simulink library "Ventilation_AIV"  (Simulink 8.2)
settings: Solver=ode45  StartTime=0.0  StopTime=10.0  RelTol=1e-3
libraries: carnot x3
settings Model: Creator=lena.frank  LastModifiedBy=drhf

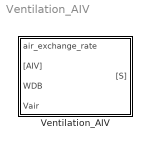
== system Ventilation_AIV ==
  Ventilation_AIV : Subsystem  mask(ACTIVE COMPONENT){co2=400}
      mask prompts: co2 "CO2 content of air in ppm"
      mask help:
      | This block represents the AIR VENTILATION from outdoors into a zone.
      |
      | r : rate of nominal air flow between outdoors and indoor, [0,1]
      | [S] : vector for sinks and sources.
      |
      | NOTE: Mass flows of water and CO2 are taken into consideration.
      |
      | ASSUMPTION:
      | Incoming air volume flow is identical to outgoing air volume flow.
      mask init:
      | CO2norm = co2*1e-6;
      mask Help: web(fullfile(path_carnot('help'),'Ventilation_AIV.html'),'-helpbrowser')
      mask Display:
      | plot([0.2 0.35], [0.8 0.7])
      | plot([0.35 0.65], [0.7 0.7])
      | plot([0.65 0.8], [0.7 0.8])
      | plot([0.65 0.8], [0.76 0.8])
      | plot([0.7 0.8], [0.65 0.8])
      | 
      | plot([0.2 0.35], [0.2 0.3])
      | plot([0.35 0.65], [0.3 0.3])
      | plot([0.65 0.8], [0.3 0.2])
      | plot([0.2 0.25], [0.2 0.32])
      | plot([0.2 0.35], [0.2 0.23])
      | 
      | plot ([0.45 0.45], [0 1])
      | plot ([0.55 0.55], [0 1])
      | 
      | plot ([0.45 0.55], [0.2 0.2])
      | plot ([0.45 0.55], [0.8 0.8])
      | 
      | plot ([0.45 0.55], [0 0.2])
      | plot ([0.45 0.55], [0.8 1])

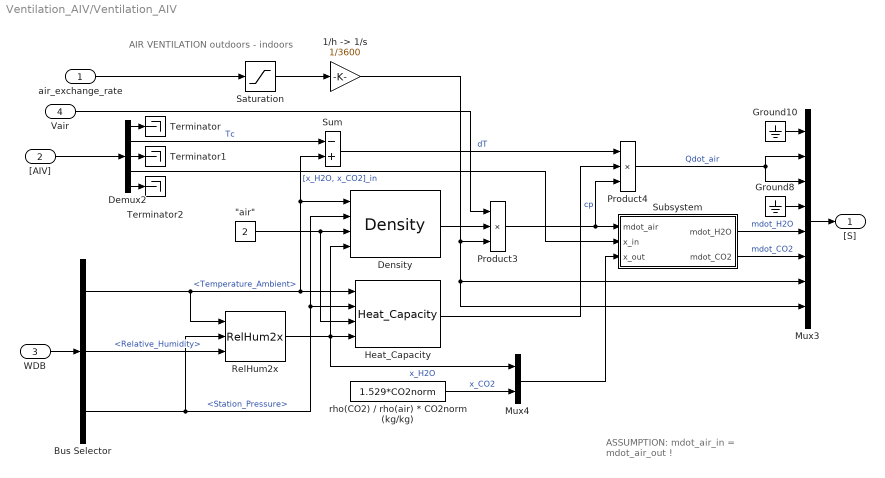
== system Ventilation_AIV/Ventilation_AIV ==
  note: AIR VENTILATION outdoors - indoors
  note: ASSUMPTION: mdot_air_in = mdot_air_out !
  air_exchange_rate : Inport
  "[AIV]" : Inport  Port=2
  WDB : Inport  Port=3
  Vair : Inport  Port=4
  "\"air\"" : Constant  Value=2
  "1/h -> 1/s" : Gain  Gain=1/3600  SaturateOnIntegerOverflow=on  OutDataTypeStr=Inherit: Same as input  ParamDataTypeStr=Inherit: Same as input
  Bus Selector : BusSelector  OutputSignals=Temperature_Ambient,Relative_Humidity,Station_Pressure
  Demux2 : Demux  Outputs=[1 1 1 2 4]
  Density : carnot/Basic/Material_Properties/Density  VariantControl=CarlibClassic  INPUTARGUMENTS=state variables (classic)  DEBUGLEVEL=DEBUGLEVEL  MAXTOTALWARNINGS=inf  MAXCONSECUTIVEWARNINGS=inf  WRITETOFILE=0  FILENAME='errors.txt'
  Ground10 : Ground
  Ground8 : Ground
  Heat_Capacity : carnot/Basic/Material_Properties/Heat_Capacity  VariantControl=CarlibClassic  INPUTARGUMENTS=state variables (classic)  DEBUGLEVEL=DEBUGLEVEL  MAXTOTALWARNINGS=inf  MAXCONSECUTIVEWARNINGS=inf  WRITETOFILE=0  FILENAME='errors.txt'
  Mux3 : Mux  Inputs=[5 1 1 2 1 1 1 1]
  Mux4 : Mux  Inputs=2
  Product3 : Product  Inputs=3  SaturateOnIntegerOverflow=on  InputSameDT=on  OutDataTypeStr=Inherit: Same as first input
  Product4 : Product  Inputs=3  SaturateOnIntegerOverflow=on  InputSameDT=on  OutDataTypeStr=Inherit: Same as first input
  RelHum2x : carnot/Basic/Material_Properties/RelHum2x
  Saturation : Saturate  UpperLimit=inf  LowerLimit=0
  Subsystem : Subsystem
  Sum : Sum  Inputs=-+  SaturateOnIntegerOverflow=on  InputSameDT=on  OutDataTypeStr=Inherit: Same as first input
  Terminator : Terminator
  Terminator1 : Terminator
  Terminator2 : Terminator
  rho(CO2) / rho(air) * CO2norm (kg/kg) : Constant  Value=1.529*CO2norm
  "[S]" : Outport
  wires:
  "1/h -> 1/s"/1 -> Product3/3, Mux3/8, Mux3/7
  Saturation/1 -> "1/h -> 1/s"/1
  Product3/1 -> Subsystem/1(mdot_air), Product4/3
  Heat_Capacity/1 -> Product4/2  "cp"
  Demux2/1 -> Terminator/1
  Sum/1 -> Product4/1  "dT"
  rho(CO2) / rho(air) * CO2norm (kg/kg)/1 -> Mux4/2  "x_CO2"
  Mux4/1 -> Subsystem/3(x_out)
  Demux2/2 -> Sum/1  "Tc"
  Demux2/3 -> Terminator1/1
  Demux2/5 -> Terminator2/1
  Demux2/4 -> Subsystem/2(x_in)  "[x_H2O, x_CO2]_in"
  "\"air\""/1 -> Density/3, Heat_Capacity/3
  RelHum2x/1 -> Mux4/1, Density/4, Heat_Capacity/4  "x_H2O"
  Bus Selector/1 -> Sum/2, Density/1, Heat_Capacity/1, RelHum2x/1  "<Temperature_Ambient>"
  Bus Selector/2 -> RelHum2x/3  "<Relative_Humidity>"
  Bus Selector/3 -> Density/2, Heat_Capacity/2, RelHum2x/2  "<Station_Pressure>"
  Density/1 -> Product3/2
  "[AIV]"/1 -> Demux2/1
  air_exchange_rate/1 -> Saturation/1
  WDB/1 -> Bus Selector/1
  Subsystem/1(mdot_H2O) -> Mux3/5  "mdot_H2O"
  Subsystem/2(mdot_CO2) -> Mux3/6  "mdot_CO2"
  Ground8/1 -> Mux3/4
  Ground10/1 -> Mux3/1
  Product4/1 -> Mux3/2, Mux3/3  "Qdot_air"
  Mux3/1 -> "[S]"/1
  Vair/1 -> Product3/1

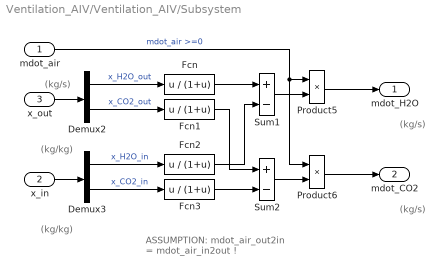
== system Ventilation_AIV/Ventilation_AIV/Subsystem ==
  note: ASSUMPTION: mdot_air_out2in = mdot_air_in2out !
  note: (kg/kg)
  note: (kg/kg)
  note: (kg/s)
  note: (kg/s)
  note: (kg/s)
  mdot_air : Inport
  x_in : Inport  Port=2
  x_out : Inport  Port=3
  Demux2 : Demux  Outputs=2
  Demux3 : Demux  Outputs=2
  Fcn{,1..3} (4 alike) : Fcn  Expr=u / (1+u)
  Product5 : Product  SaturateOnIntegerOverflow=on  InputSameDT=on  OutDataTypeStr=Inherit: Same as first input
  Product6 : Product  SaturateOnIntegerOverflow=on  InputSameDT=on  OutDataTypeStr=Inherit: Same as first input
  Sum1 : Sum  Inputs=+-  SaturateOnIntegerOverflow=on  InputSameDT=on  OutDataTypeStr=Inherit: Same as first input
  Sum2 : Sum  Inputs=+-  SaturateOnIntegerOverflow=on  InputSameDT=on  OutDataTypeStr=Inherit: Same as first input
  mdot_H2O : Outport
  mdot_CO2 : Outport  Port=2
  wires:
  Product5/1 -> mdot_H2O/1
  Product6/1 -> mdot_CO2/1
  mdot_air/1 -> Product5/1, Product6/1  "mdot_air >=0"
  Sum1/1 -> Product5/2
  Sum2/1 -> Product6/2
  Fcn3/1 -> Sum2/2
  Fcn1/1 -> Sum2/1
  Fcn2/1 -> Sum1/2
  Fcn/1 -> Sum1/1
  x_in/1 -> Demux3/1
  Demux3/1 -> Fcn2/1  "x_H2O_in"
  Demux3/2 -> Fcn3/1  "x_CO2_in"
  Demux2/2 -> Fcn1/1  "x_CO2_out"
  Demux2/1 -> Fcn/1  "x_H2O_out"
  x_out/1 -> Demux2/1
